simulink model "frt_statcom"  (R2025a)
settings: Solver=ode23tb  StartTime=0.0  StopTime=0.8  RelTol=1e-3
libraries: spsSeriesRLCBranchLib x2, spsThreePhaseVIMeasurementLib x2, spsIGBTLib x1, spsThreePhaseSourceLib x1, spsThreePhaseFaultLib x1, spsThreePhaseSeriesRLCBranchLib x1, spsThreePhaseSeriesRLCLoadLib x1, spsVoltageMeasurementLib x1, spsUniversalBridgeLib x1, sps_lib x1
settings Model: Creator=m1391  LastModifiedBy=m1391

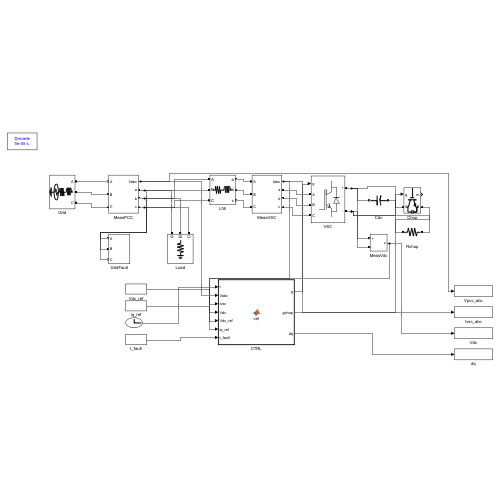
[thumbnail: Simulink's stored preview of the top-level diagram]
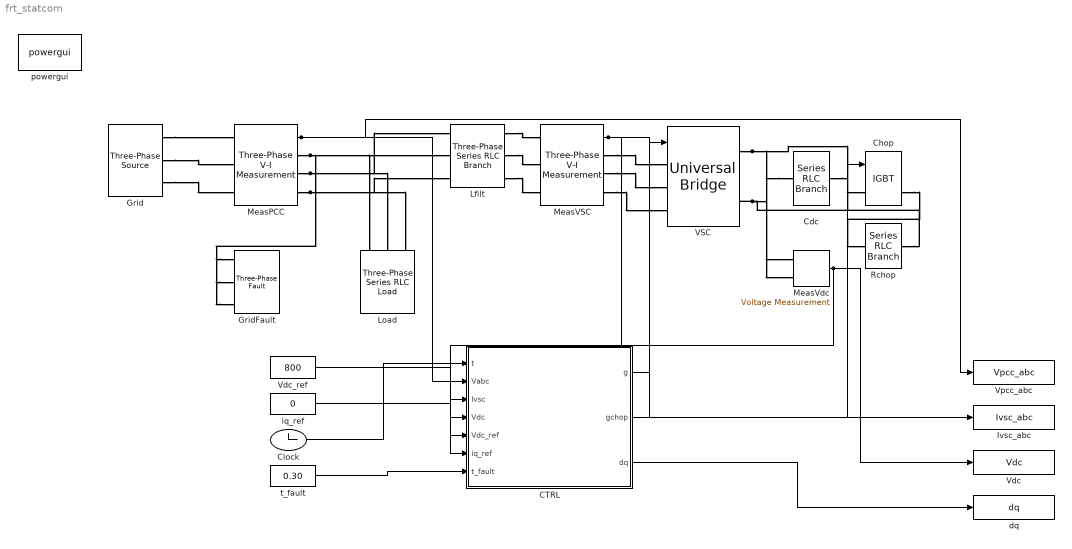
== system frt_statcom ==
  CTRL : MATLAB Function  TreatAsAtomicUnit=on
  Cdc : spsSeriesRLCBranchLib/Series RLC Branch  LConnTagsString=__new0  RConnTagsString=__new0  BranchType=C  Resistance=1  Inductance=1e-3  SetiL0=off  InitialCurrent=0  Capacitance=0.0022  Setx0=on  InitialVoltage=800  Measurements=None
  Chop : spsIGBTLib/IGBT  Ron=0.001  Lon=0  Vf=1  Tf=1e-6  Tt=2e-6  IC=0  Rs=1e5  Cs=inf  Measurements=on
  Clock : Clock
  Grid : spsThreePhaseSourceLib/Three-Phase Source  InternalConnection=Yg  VoltagePhases=off  Voltage=400  PhaseAngle=0  Voltage_phases=[25e3 25e3 25e3]/sqrt(3)  PhaseAngles_phases=[0 -120 +120]  Frequency=50  NonIdealSource=on  SpecifyImpedance=off  Resistance=0.019  Inductance=0.42e-3  ShortCircuitLevel=100e6  BaseVoltage=25e3  XRratio=7  BusType=swing  Pref=10e3  Qref=0  Prefabc=[10e3, 10e3, 10e3]  Qrefabc=[0, 0, 0]  Qmin=-inf  Qmax=inf
  GridFault : spsThreePhaseFaultLib/Three-Phase Fault  InitialStates=0  FaultA=off  FaultB=off  FaultC=off  GroundFault=off  SwitchTimes=[99 100]  External=off  SwitchStatus=NaN  FaultResistance=0.15  GroundResistance=0.001  SnubberResistance=1e6  SnubberCapacitance=inf  Measurements=None
  Ivsc_abc : ToWorkspace  VariableName=Ivsc_abc  SampleTime=5e-05
  Lfilt : spsThreePhaseSeriesRLCBranchLib/Three-Phase Series RLC Branch  LConnTagsString=A|B|C  RConnTagsString=A|B|C  BranchType=RL  Resistance=0.05  Inductance=0.003  Capacitance=1e-6  Measurements=None
  Load : spsThreePhaseSeriesRLCLoadLib/Three-Phase Series RLC Load  LConnTagsString=A|B|C  Configuration=Y (grounded)  NominalVoltage=400  Vabc=[1e3 1e3 1e3]  Vabcp=[1e3 1e3 1e3]  NominalFrequency=50  UnbalancedPower=off  ActivePower=400000  InductivePower=0  CapacitivePower=0  Pabc=[10e3 9e3 11e3]  QLabc=[100 90 110]  QCabc=[100 90 110]  Pabcp=[10e3 9e3 11e3]  QLabcp=[100 90 110]  QCabcp=[100 90 110]  Measurements=None  LoadType=constant Z
  MeasPCC : spsThreePhaseVIMeasurementLib/Three-Phase V-I Measurement  VoltageMeasurement=phase-to-ground  SetLabelV=off  LabelV=Vabc  Vpu=off  VpuLL=off  CurrentMeasurement=no  SetLabelI=off  LabelI=Iabc  Ipu=off  Pbase=100e6  Vbase=500e3  OutputType=Complex  PhasorSimulation=off  PSBequivalent=0
  MeasVSC : spsThreePhaseVIMeasurementLib/Three-Phase V-I Measurement  VoltageMeasurement=no  SetLabelV=off  LabelV=Vabc  Vpu=off  VpuLL=off  CurrentMeasurement=yes  SetLabelI=off  LabelI=Iabc  Ipu=off  Pbase=100e6  Vbase=500e3  OutputType=Complex  PhasorSimulation=off  PSBequivalent=0
  MeasVdc : spsVoltageMeasurementLib/Voltage Measurement  PhasorSimulation=off  OutputType=Complex  PSBequivalent=0
  Rchop : spsSeriesRLCBranchLib/Series RLC Branch  LConnTagsString=__new0  RConnTagsString=__new0  BranchType=R  Resistance=5.33  Inductance=1e-3  SetiL0=off  InitialCurrent=0  Capacitance=1e-6  Setx0=off  InitialVoltage=0  Measurements=None
  VSC : spsUniversalBridgeLib/Universal Bridge  Arms=3  SnubberResistance=1e5  SnubberCapacitance=inf  Device=IGBT / Diodes  Ron=1e-3  Lon=0  ForwardVoltages="[  0  0  ]"  ForwardVoltage=0  GTOparameters=[ 10e-6 , 20e-6 ]  IGBTparameters=[ 1e-6 , 2e-6 ]  Measurements=None  Measurements_2=None  converterType=Rectifier
  Vdc : ToWorkspace  VariableName=Vdc  SampleTime=5e-05
  Vdc_ref : Constant  Value=800
  Vpcc_abc : ToWorkspace  VariableName=Vpcc_abc  SampleTime=5e-05
  dq : ToWorkspace  VariableName=dq  SampleTime=5e-05
  iq_ref : Constant  Value=0
  powergui : sps_lib/powergui  Priority=1  SimulationMode=Discrete  SampleTime=5e-05  frequency=60  Iterations=50  frequencyindice=50  Pbase=100e6  ErrMax=1e-4  UnitsV=kV  UnitsW=MW  buscounter=0  FunctionMessages=off  echomessages=off  EnableUseOfTLC=off  CurrentSourceSwitches=off  DisableSnubberDevices=off  DisableRonSwitches=off  DisableVfSwitches=off  DisplayEquations=off  AutomaticDiscreteSolvers=off  SolverType=Tustin/Backward Euler (TBE)  Interpol=off  ExternalGateDelay=off  methode=off  Ts=100  x0status=blocks  SPID=on  SwTol=0  HookPort=off  NonlinearTolerance=1e-4  nMaxIteration=100  ContinueOnMaxIteration=off  RestoreLinks=warning  ResistiveCurrentMeasurement=off  Frange=[0:2:500]  Ylog=off  Xlog=on  ShowGrid=off  save=off  variable=ZData  structure=0  ZoomFFT=off  StartTime=0.0  cycles=1  DisplayStyle=1  fundamental=60  FreqAxis=off  MaxFrequency=1000  frequencyindicesteady=1  RmsSteady=1  display=off
  t_fault : Constant  Value=0.30
  wires:
  MeasPCC/1 -> Vpcc_abc/1, CTRL/2(Vabc)
  MeasVSC/1 -> Ivsc_abc/1, CTRL/3(Ivsc)
  MeasVdc/1 -> Vdc/1, CTRL/4(Vdc)
  Clock/1 -> CTRL/1(t)
  Vdc_ref/1 -> CTRL/5(Vdc_ref)
  iq_ref/1 -> CTRL/6(iq_ref)
  t_fault/1 -> CTRL/7(t_fault)
  CTRL/1(g) -> VSC/1
  CTRL/2(gchop) -> Chop/1
  CTRL/3(dq) -> dq/1
  connections:
  Grid/RConn1 -- MeasPCC/LConn1
  GridFault/LConn1 -- MeasPCC/RConn1 -- Load/LConn1 -- Lfilt/LConn1
  Lfilt/RConn1 -- MeasVSC/LConn1
  MeasVSC/RConn1 -- VSC/LConn1
  Grid/RConn2 -- MeasPCC/LConn2
  GridFault/LConn2 -- MeasPCC/RConn2 -- Load/LConn2 -- Lfilt/LConn2
  Lfilt/RConn2 -- MeasVSC/LConn2
  MeasVSC/RConn2 -- VSC/LConn2
  Grid/RConn3 -- MeasPCC/LConn3
  GridFault/LConn3 -- MeasPCC/RConn3 -- Load/LConn3 -- Lfilt/LConn3
  Lfilt/RConn3 -- MeasVSC/LConn3
  MeasVSC/RConn3 -- VSC/LConn3
  Cdc/LConn1 -- VSC/RConn1 -- MeasVdc/LConn1 -- Chop/LConn1
  Cdc/RConn1 -- MeasVdc/LConn2 -- VSC/RConn2 -- Rchop/RConn1
  Chop/RConn1 -- Rchop/LConn1

== matlab function frt_statcom/CTRL ==
  data: t input; g output; Vabc input; Ivsc input; Vdc input; Vdc_ref input; iq_ref input; t_fault input; gchop output; dq output
function [g, gchop, dq] = ctrl(t, Vabc, Ivsc, Vdc, Vdc_ref, iq_ref, t_fault)
%#codegen
persistent th wint idi iqi vdi tprev en idr
if isempty(th) || t < 1e-9
    th = 0; wint = 0; idi = 0; iqi = 0; vdi = 0; tprev = 0; en = 0; idr = 0;
end
if Vdc > 620; en = 1; end   % latch control ON once DC bus precharged
dt = t - tprev; if dt < 0; dt = 0; end; if dt > 1e-3; dt = 1e-3; end; tprev = t;
w0 = 2*pi*50; Lsh = 3e-3; Imax = 173.2;
Va=Vabc(1); Vb=Vabc(2); Vc=Vabc(3);
Valpha = (2/3)*(Va - 0.5*Vb - 0.5*Vc);
Vbeta  = (2/3)*(sqrt(3)/2)*(Vb - Vc);
% --- dq-PLL: drive Vq->0 ---
Vd =  cos(th)*Valpha + sin(th)*Vbeta;
Vq = -sin(th)*Valpha + cos(th)*Vbeta;
Vm = sqrt(Vd*Vd + Vq*Vq); if Vm < 100; Vm = 100; end
err = Vq / Vm;
Kp_pll = 90; Ki_pll = 1500;
wint = wint + Ki_pll*err*dt; if wint>150; wint=150; elseif wint<-150; wint=-150; end
w = w0 + Kp_pll*err + wint;
th = th + w*dt; th = mod(th, 2*pi);
% --- VSC current in dq (load convention: current INTO VSC from bus) ---
Ia=Ivsc(1); Ib=Ivsc(2); Ic=Ivsc(3);
Ialpha=(2/3)*(Ia-0.5*Ib-0.5*Ic); Ibeta=(2/3)*(sqrt(3)/2)*(Ib-Ic);
id =  cos(th)*Ialpha + sin(th)*Ibeta;
iq = -sin(th)*Ialpha + cos(th)*Ibeta;
% --- outer Vdc PI -> active current ref (charges DC); rate- & range-limited ---
Kpv = 0.50; Kiv = 8.0;
ev = (Vdc_ref - Vdc)/Vdc_ref;
vdi = vdi + Kiv*ev*dt; if vdi>1.0; vdi=1.0; elseif vdi<-1.0; vdi=-1.0; end
idtgt = (Kpv*ev + vdi) * Imax;
if idtgt > 0.9*Imax; idtgt = 0.9*Imax; elseif idtgt < -0.9*Imax; idtgt = -0.9*Imax; end
% rate-limit id_ref so the inner loop never sees a huge step (avoids saturation)
dmax = 4000*dt;
dstep = idtgt - idr; if dstep>dmax; dstep=dmax; elseif dstep<-dmax; dstep=-dmax; end
idr = idr + dstep;
% --- reactive-priority current limit ---
iqr = iq_ref; if iqr>0.3*Imax; iqr=0.3*Imax; elseif iqr<-0.3*Imax; iqr=-0.3*Imax; end
idm = sqrt(max(0, Imax*Imax - iqr*iqr));
if idr<-idm; idr=-idm; elseif idr>idm; idr=idm; end
% --- dq current PI + decoupling + grid feedforward (gentler Kp; anti-windup) ---
Kp = 2.5; Ki = 150.0;
ed = idr - id; eq = iqr - iq;
ud = Vd - (Kp*ed + idi) + w0*Lsh*iq;
uq = Vq - (Kp*eq + iqi) - w0*Lsh*id;
% --- modulation (fraction of Vdc/2) ---
half = max(50, Vdc/2);
md = ud/half; mq = uq/half;
sat = (abs(md)>1) || (abs(mq)>1);
if ~sat
    idi = idi + Ki*ed*dt; iqi = iqi + Ki*eq*dt;
    if idi>300; idi=300; elseif idi<-300; idi=-300; end
    if iqi>300; iqi=300; elseif iqi<-300; iqi=-300; end
end
ma = md*cos(th)        - mq*sin(th);
mb = md*cos(th-2*pi/3) - mq*sin(th-2*pi/3);
mc = md*cos(th+2*pi/3) - mq*sin(th+2*pi/3);
if ma>1; ma=1; elseif ma<-1; ma=-1; end
if mb>1; mb=1; elseif mb<-1; mb=-1; end
if mc>1; mc=1; elseif mc<-1; mc=-1; end
% --- SPWM gates (fc = 5 kHz) ---
fc = 5000; carrier = 2*abs(2*(fc*t - floor(fc*t+0.5))) - 1;
ga = ma>=carrier; gb = mb>=carrier; gc = mc>=carrier;
g = double([ga; ~ga; gb; ~gb; gc; ~gc]);
% --- soft-start precharge: gates OFF (diode rectify) until latched ON ---
if en < 0.5
    g = zeros(6,1); idi = 0; iqi = 0; vdi = 0;
end
% --- conditional DC chopper: engage above 1.20 pu (fault overvoltage only) ---
gchop = double(Vdc > 1.20*800);
dq = [id; iq; idr; iqr; Vd; Vm; th];
